simulink model "sim_DOB_vs_UIO"  (R2020b)
settings: Solver=FixedStepAuto  StartTime=0.0  StopTime=0.5  FixedStep=0.0001  RelTol=1e-3
values from neighbouring files (symbols this model uses):
  A_dob = [A E;0 0 1]    [DOB_vs_UIO.m]
  A_hat = A - L1*C*A_til - L2*C    [DOB_vs_UIO.m]
  Ac = [0 1;-c_th/J -k/J ]    [DOB_vs_UIO.m]
  B_dob = [B;0]    [DOB_vs_UIO.m]
  B_hat = B - L1*C*B_til    [DOB_vs_UIO.m]
  Bc = [0;1/J]    [DOB_vs_UIO.m]
  C = [1 0]    [DOB_vs_UIO.m]
  C_dob = [C 0]    [DOB_vs_UIO.m]
  Ec = [0;1/J]    [DOB_vs_UIO.m]
  i = 0.5    [DOB_vs_UIO.m]
  invCE_til = inv(C*E_til)    [DOB_vs_UIO.m]
  L1 = E * invCE_til    [DOB_vs_UIO.m]
  L2 = place((A - L1*C*A_til)', C', pole_uio)'    [DOB_vs_UIO.m]
  L_dob = place(A_dob', C_dob', pole_dob)'    [DOB_vs_UIO.m]
  T = 0.001    [DOB_vs_UIO.m]
undefined symbols (not defined in the file or in its folder): A_til, B_til
settings Model: Creator=s0612  LastModifiedBy=s0612

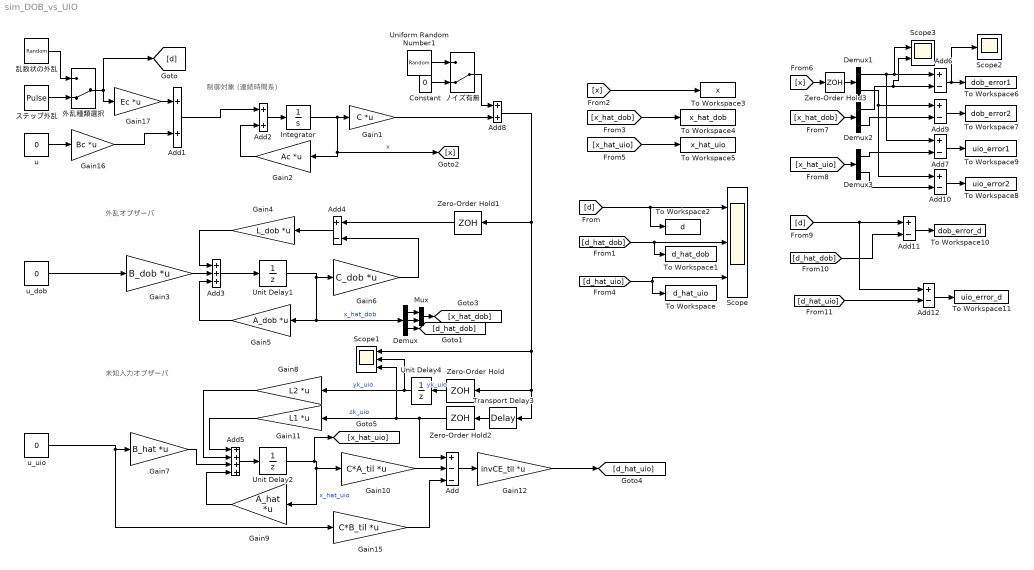
== system sim_DOB_vs_UIO ==
  note: 外乱オブザーバ
  note: 制御対象 (連続時間系)
  note: 未知入力オブザーバ
  Add : Sum  Inputs=+--
  Add1 : Sum
  Add{4,6..7,9..12} (7 alike) : Sum  Inputs=+-
  Add2 : Sum
  Add3 : Sum  Inputs=+++
  Add5 : Sum  Inputs=++++
  Add8 : Sum
  Constant : Constant  Value=0
  Demux : Demux  Outputs=3
  Demux1 : Demux  Outputs=2
  Demux2 : Demux  Outputs=2
  Demux3 : Demux  Outputs=2
  Gain1 : Gain  Gain=C  Multiplication=Matrix(K*u) (u vector)
  Gain10 : Gain  Gain=C*A_til  Multiplication=Matrix(K*u) (u vector)
  Gain11 : Gain  Gain=L1  Multiplication=Matrix(K*u) (u vector)
  Gain12 : Gain  Gain=invCE_til  Multiplication=Matrix(K*u) (u vector)
  Gain15 : Gain  Gain=C*B_til  Multiplication=Matrix(K*u) (u vector)
  Gain16 : Gain  Gain=Bc  Multiplication=Matrix(K*u) (u vector)
  Gain17 : Gain  Gain=Ec  Multiplication=Matrix(K*u) (u vector)
  Gain2 : Gain  Gain=Ac  Multiplication=Matrix(K*u) (u vector)
  Gain3 : Gain  Gain=B_dob  Multiplication=Matrix(K*u) (u vector)
  Gain4 : Gain  Gain=L_dob  Multiplication=Matrix(K*u) (u vector)
  Gain5 : Gain  Gain=A_dob  Multiplication=Matrix(K*u) (u vector)
  Gain6 : Gain  Gain=C_dob  Multiplication=Matrix(K*u) (u vector)
  Gain7 : Gain  Gain=B_hat  Multiplication=Matrix(K*u) (u vector)
  Gain8 : Gain  Gain=L2  Multiplication=Matrix(K*u) (u vector)
  Gain9 : Gain  Gain=A_hat  Multiplication=Matrix(K*u) (u vector)
  Integrator : Integrator
  Mux : Mux  Inputs=2
  Scope : Scope  NumInputPorts=3
  Scope1 : Scope  NumInputPorts=3
  Scope2 : Scope
  Scope3 : Scope  NumInputPorts=2
  To Workspace : ToWorkspace  VariableName=d_hat_uio  SaveFormat=Timeseries  SampleTime=-1
  To Workspace1 : ToWorkspace  VariableName=d_hat_dob  SaveFormat=Timeseries  SampleTime=-1
  To Workspace10 : ToWorkspace  VariableName=dob_error_d  SaveFormat=Timeseries  SampleTime=-1
  To Workspace11 : ToWorkspace  VariableName=uio_error_d  SaveFormat=Timeseries  SampleTime=-1
  To Workspace2 : ToWorkspace  VariableName=d  SaveFormat=Timeseries  SampleTime=-1
  To Workspace3 : ToWorkspace  VariableName=x  SaveFormat=Timeseries  SampleTime=-1
  To Workspace4 : ToWorkspace  VariableName=x_hat_dob  SaveFormat=Timeseries  SampleTime=-1
  To Workspace5 : ToWorkspace  VariableName=x_hat_uio  SaveFormat=Timeseries  SampleTime=-1
  To Workspace6 : ToWorkspace  VariableName=dob_error1  SaveFormat=Timeseries  SampleTime=-1
  To Workspace7 : ToWorkspace  VariableName=dob_error2  SaveFormat=Timeseries  SampleTime=-1
  To Workspace8 : ToWorkspace  VariableName=uio_error2  SaveFormat=Timeseries  SampleTime=-1
  To Workspace9 : ToWorkspace  VariableName=uio_error1  SaveFormat=Timeseries  SampleTime=-1
  Transport Delay3 : TransportDelay  DelayTime=(1-i)*T
  Uniform Random Number1 : UniformRandomNumber  Minimum=-0.00001  Maximum=0.00001  Seed=1  SampleTime=0.01
  Unit Delay1 : UnitDelay  SampleTime=T  HasFrameUpgradeWarning=on
  Unit Delay2 : UnitDelay  SampleTime=T  HasFrameUpgradeWarning=on
  Unit Delay4 : UnitDelay  SampleTime=-1  HasFrameUpgradeWarning=on
  Zero-Order Hold{,1..3} (4 alike) : ZeroOrderHold  SampleTime=T
  u : Constant  Value=0
  u_dob : Constant  Value=0
  u_uio : Constant  Value=0
  ステップ外乱 : DiscretePulseGenerator  PulseType=Time based  Period=0.5  PulseWidth=50  PhaseDelay=0.1
  ノイズ有無 : ManualSwitch  CurrentSetting=0
  乱数状の外乱 : UniformRandomNumber  SampleTime=0.01
  外乱種類選択 : ManualSwitch  CurrentSetting=0
  wires:
  外乱種類選択/1 -> [d], Gain17/1
  Add2/1 -> Integrator/1
  Add1/1 -> Add2/1
  Gain2/1 -> Add2/2
  Add3/1 -> Unit Delay1/1
  Add4/1 -> Gain4/1
  Gain3/1 -> Add3/2
  Gain5/1 -> Add3/3
  Unit Delay1/1 -> Gain6/1, Demux/1, Gain5/1  "x_hat_dob"
  [d] -> To Workspace2/1, Scope/1
  Integrator/1 -> [x], Gain2/1, Gain1/1  "x"
  Gain4/1 -> Add3/1
  Demux/3 -> [d_hat_dob]
  [d_hat_dob] -> To Workspace1/1, Scope/2
  Demux/1 -> Mux/1
  Demux/2 -> Mux/2
  Mux/1 -> [x_hat_dob]
  u/1 -> Gain16/1
  u_dob/1 -> Gain3/1
  Unit Delay2/1 -> Gain9/1, Gain10/1, [x_hat_uio]  "x_hat_uio"
  Gain6/1 -> Add4/2
  u_uio/1 -> Gain15/1, Gain7/1
  Gain8/1 -> Add5/2
  Gain11/1 -> Add5/1
  Zero-Order Hold2/1 -> Scope1/3, Gain11/1, Add/1  "zk_uio"
  Zero-Order Hold1/1 -> Add4/1
  Gain9/1 -> Add5/4
  Gain7/1 -> Add5/3
  Add/1 -> Gain12/1
  [d_hat_uio] -> To Workspace/1, Scope/3
  Gain15/1 -> Add/3
  Gain16/1 -> Add1/2
  Gain17/1 -> Add1/1
  Gain10/1 -> Add/2
  Add5/1 -> Unit Delay2/1
  Zero-Order Hold/1 -> Unit Delay4/1  "yk_uio"
  Uniform Random Number1/1 -> ノイズ有無/1
  Gain1/1 -> Add8/2
  Constant/1 -> ノイズ有無/2
  ノイズ有無/1 -> Add8/1
  ステップ外乱/1 -> 外乱種類選択/2
  乱数状の外乱/1 -> 外乱種類選択/1
  Gain12/1 -> [d_hat_uio]
  [x] -> To Workspace3/1
  [x_hat_dob] -> To Workspace4/1
  [x_hat_uio] -> To Workspace5/1
  Add8/1 -> Zero-Order Hold1/1, Zero-Order Hold/1, Transport Delay3/1, Scope1/1
  Transport Delay3/1 -> Zero-Order Hold2/1
  Unit Delay4/1 -> Scope1/2, Gain8/1  "yk_uio"
  [x_hat_dob] -> Demux2/1
  [x_hat_uio] -> Demux3/1
  Demux3/1 -> Add7/2
  Add6/1 -> Scope2/1, To Workspace6/1
  Add7/1 -> To Workspace9/1
  Demux2/2 -> Add9/2
  Add9/1 -> To Workspace7/1
  Demux3/2 -> Add10/2
  Add10/1 -> To Workspace8/1
  Add11/1 -> To Workspace10/1
  [d_hat_dob] -> Add11/2
  Add12/1 -> To Workspace11/1
  [d_hat_uio] -> Add12/2
  [x] -> Zero-Order Hold3/1
  Demux2/1 -> Scope3/2, Add6/2
  Zero-Order Hold3/1 -> Demux1/1
  Demux1/1 -> Add7/1, Add6/1, Scope3/1
  Demux1/2 -> Add10/1, Add9/1
  [d] -> Add12/1, Add11/1
